simulink model "wiener"  (R2019b)
settings: Solver=VariableStepAuto  StartTime=0.0  StopTime=stopTime  RelTol=1e-3
InitFcn:
  | Init;
values from neighbouring files (symbols this model uses):
  Ts = 1/Fs    [Init.m]
libraries: simulink x2
settings Model: Creator=cb54103  LastModifiedBy=cb54103

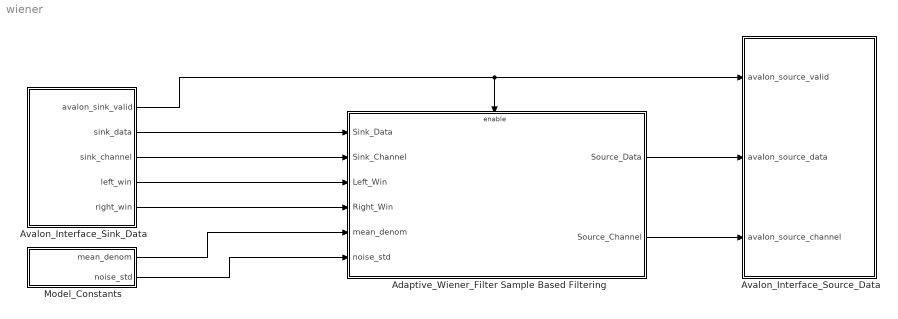
== system wiener ==
  Adaptive_Wiener_Filter Sample Based Filtering : Subsystem
  Avalon_Interface_Sink_Data : Subsystem
  Avalon_Interface_Source_Data : Subsystem
  Model_Constants : Subsystem
  wires:
  Adaptive_Wiener_Filter Sample Based Filtering/1(Source_Data) -> Avalon_Interface_Source_Data/2(avalon_source_data)
  Adaptive_Wiener_Filter Sample Based Filtering/2(Source_Channel) -> Avalon_Interface_Source_Data/3(avalon_source_channel)
  Avalon_Interface_Sink_Data/2(sink_data) -> Adaptive_Wiener_Filter Sample Based Filtering/1(Sink_Data)
  Avalon_Interface_Sink_Data/3(sink_channel) -> Adaptive_Wiener_Filter Sample Based Filtering/2(Sink_Channel)
  Avalon_Interface_Sink_Data/4(left_win) -> Adaptive_Wiener_Filter Sample Based Filtering/3(Left_Win)
  Avalon_Interface_Sink_Data/5(right_win) -> Adaptive_Wiener_Filter Sample Based Filtering/4(Right_Win)
  Avalon_Interface_Sink_Data/1(avalon_sink_valid) -> Adaptive_Wiener_Filter Sample Based Filtering/Enable, Avalon_Interface_Source_Data/1(avalon_source_valid)
  Model_Constants/1(mean_denom) -> Adaptive_Wiener_Filter Sample Based Filtering/5(mean_denom)
  Model_Constants/2(noise_std) -> Adaptive_Wiener_Filter Sample Based Filtering/6(noise_std)

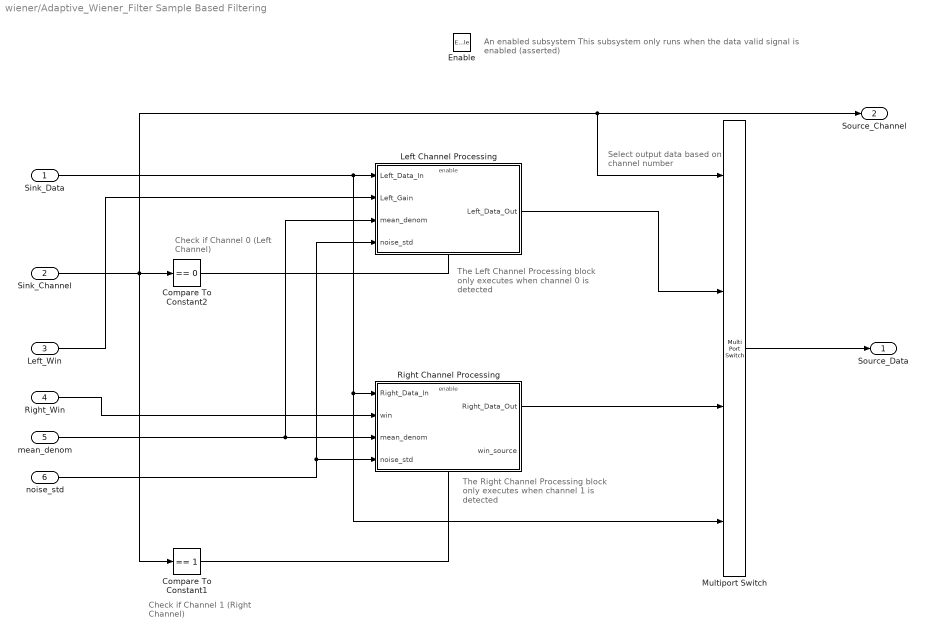
== system wiener/Adaptive_Wiener_Filter Sample Based Filtering ==
  note: The Left Channel Processing block
      | only executes when channel 0
      | is detected
  note: The Right Channel Processing block
      | only executes when channel 1
      | is detected
  note: Check if Channel 1
      | (Right Channel)
  note: Check if Channel 0
      | (Left Channel)
  note: Select output data
      | based on channel number
  note: An enabled subsystem
      | This subsystem only runs when the data valid signal is enabled (asserted)
  Sink_Data : Inport
  Sink_Channel : Inport  Port=2
  Left_Win : Inport  Port=3
  Right_Win : Inport  Port=4
  mean_denom : Inport  Port=5
  noise_std : Inport  Port=6
  Enable : EnablePort
  Compare To Constant1 : simulink/Logic and Bit Operations/Compare To Constant  relop===  const=1  OutDataTypeStr=boolean
  Compare To Constant2 : simulink/Logic and Bit Operations/Compare To Constant  relop===  const=0  OutDataTypeStr=boolean
  Left Channel Processing : Subsystem  TreatAsAtomicUnit=on
  Multiport Switch : MultiPortSwitch  DataPortOrder=Zero-based contiguous  zeroidx=on
  Right Channel Processing : Subsystem  TreatAsAtomicUnit=on
  Source_Data : Outport  InitialOutput=0  VectorParamsAs1DForOutWhenUnconnected=off
  Source_Channel : Outport  Port=2  InitialOutput=0  VectorParamsAs1DForOutWhenUnconnected=off
  wires:
  Left Channel Processing/1("Left_Data_Out ") -> Multiport Switch/2
  Multiport Switch/1 -> Source_Data/1
  Compare To Constant2/1 -> Left Channel Processing/Enable
  Right_Win/1 -> Right Channel Processing/2(win)
  Left_Win/1 -> Left Channel Processing/2(Left_Gain)
  Sink_Data/1 -> Multiport Switch/4, Right Channel Processing/1(Right_Data_In), Left Channel Processing/1(Left_Data_In)
  Right Channel Processing/1("Right_Data_Out ") -> Multiport Switch/3
  Sink_Channel/1 -> Source_Channel/1, Multiport Switch/1, Compare To Constant1/1, Compare To Constant2/1
  Compare To Constant1/1 -> Right Channel Processing/Enable
  mean_denom/1 -> Left Channel Processing/3(mean_denom), Right Channel Processing/3(mean_denom)
  noise_std/1 -> Left Channel Processing/4(noise_std), Right Channel Processing/4(noise_std)

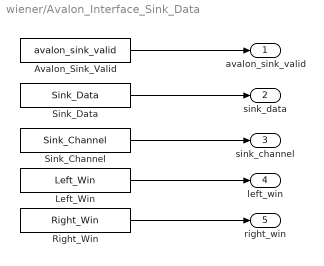
== system wiener/Avalon_Interface_Sink_Data ==
  Avalon_Sink_Valid : FromWorkspace  VariableName=avalon_sink_valid  SampleTime=Ts
  Left_Win : FromWorkspace  VariableName=Left_Win  SampleTime=Ts
  Right_Win : FromWorkspace  VariableName=Right_Win  SampleTime=Ts
  Sink_Channel : FromWorkspace  VariableName=Sink_Channel  SampleTime=Ts
  Sink_Data : FromWorkspace  VariableName=Sink_Data  SampleTime=Ts
  avalon_sink_valid : Outport  InitialOutput=0  VectorParamsAs1DForOutWhenUnconnected=off
  sink_data : Outport  Port=2  InitialOutput=0  VectorParamsAs1DForOutWhenUnconnected=off
  sink_channel : Outport  Port=3  InitialOutput=0  VectorParamsAs1DForOutWhenUnconnected=off
  left_win : Outport  Port=4  InitialOutput=0  VectorParamsAs1DForOutWhenUnconnected=off
  right_win : Outport  Port=5  InitialOutput=0  VectorParamsAs1DForOutWhenUnconnected=off
  wires:
  Sink_Channel/1 -> sink_channel/1
  Avalon_Sink_Valid/1 -> avalon_sink_valid/1
  Sink_Data/1 -> sink_data/1
  Left_Win/1 -> left_win/1
  Right_Win/1 -> right_win/1

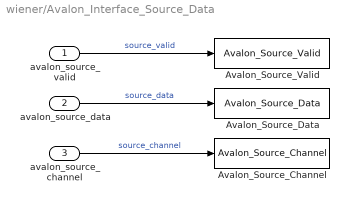
== system wiener/Avalon_Interface_Source_Data ==
  avalon_source_valid : Inport
  avalon_source_data : Inport  Port=2
  avalon_source_channel : Inport  Port=3
  Avalon_Source_Channel : ToWorkspace  VariableName=Avalon_Source_Channel  SaveFormat=Timeseries  SampleTime=-1
  Avalon_Source_Data : ToWorkspace  VariableName=Avalon_Source_Data  SaveFormat=Timeseries  SampleTime=-1
  Avalon_Source_Valid : ToWorkspace  VariableName=Avalon_Source_Valid  SaveFormat=Timeseries  SampleTime=-1
  wires:
  avalon_source_valid/1 -> Avalon_Source_Valid/1  "source_valid"
  avalon_source_data/1 -> Avalon_Source_Data/1  "source_data"
  avalon_source_channel/1 -> Avalon_Source_Channel/1  "source_channel"

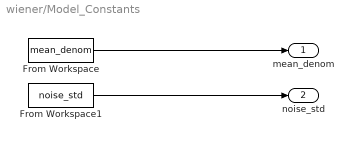
== system wiener/Model_Constants ==
  From Workspace : FromWorkspace  VariableName=mean_denom  SampleTime=Ts
  From Workspace1 : FromWorkspace  VariableName=noise_std  SampleTime=Ts
  mean_denom : Outport
  noise_std : Outport  Port=2
  wires:
  From Workspace/1 -> mean_denom/1
  From Workspace1/1 -> noise_std/1

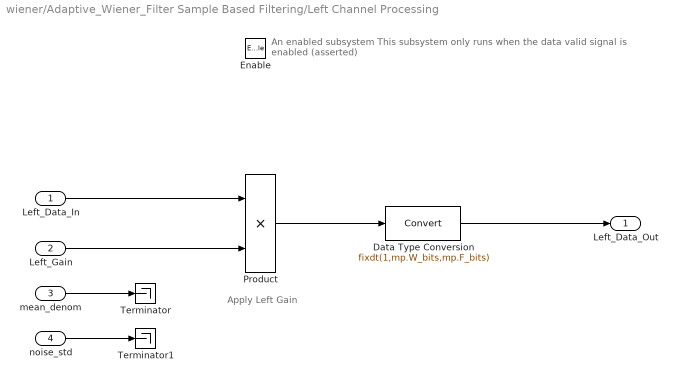
== system wiener/Adaptive_Wiener_Filter Sample Based Filtering/Left Channel Processing ==
  note: Apply Left Gain
  note: An enabled subsystem
      | This subsystem only runs when the data valid signal is enabled (asserted)
  Left_Data_In : Inport
  Left_Gain : Inport  Port=2
  mean_denom : Inport  Port=3
  noise_std : Inport  Port=4
  Enable : EnablePort
  Data Type Conversion : DataTypeConversion  OutDataTypeStr=fixdt(1,mp.W_bits,mp.F_bits)
  Product : Product
  Terminator : Terminator
  Terminator1 : Terminator
  "Left_Data_Out " : Outport  InitialOutput=0  VectorParamsAs1DForOutWhenUnconnected=off
  wires:
  Left_Data_In/1 -> Product/1
  Product/1 -> Data Type Conversion/1
  Data Type Conversion/1 -> "Left_Data_Out "/1
  Left_Gain/1 -> Product/2
  mean_denom/1 -> Terminator/1
  noise_std/1 -> Terminator1/1

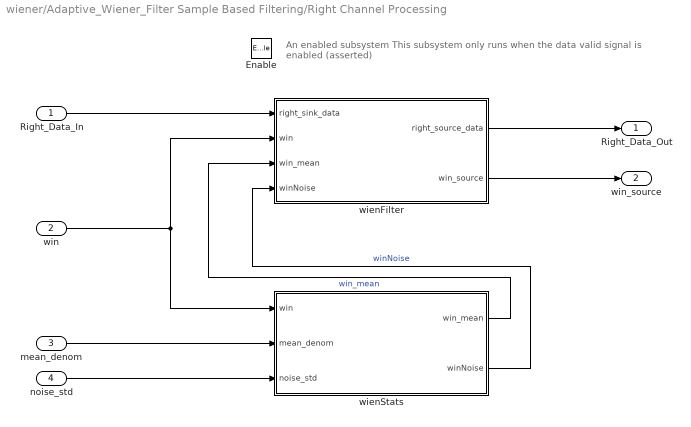
== system wiener/Adaptive_Wiener_Filter Sample Based Filtering/Right Channel Processing ==
  note: An enabled subsystem
      | This subsystem only runs when the data valid signal is enabled (asserted)
  Right_Data_In : Inport
  win : Inport  Port=2
  mean_denom : Inport  Port=3
  noise_std : Inport  Port=4
  Enable : EnablePort
  wienFilter : Subsystem
  wienStats : Subsystem
  "Right_Data_Out " : Outport  InitialOutput=0  VectorParamsAs1DForOutWhenUnconnected=off
  win_source : Outport  Port=2  InitialOutput=0  VectorParamsAs1DForOutWhenUnconnected=off
  wires:
  wienFilter/1(right_source_data) -> "Right_Data_Out "/1
  mean_denom/1 -> wienStats/2(mean_denom)
  noise_std/1 -> wienStats/3(noise_std)
  Right_Data_In/1 -> wienFilter/1(right_sink_data)
  win/1 -> wienFilter/2(win), wienStats/1(win)
  wienStats/1(win_mean) -> wienFilter/3(win_mean)  "win_mean"
  wienStats/2(winNoise) -> wienFilter/4(winNoise)  "winNoise"
  wienFilter/2(win_source) -> win_source/1

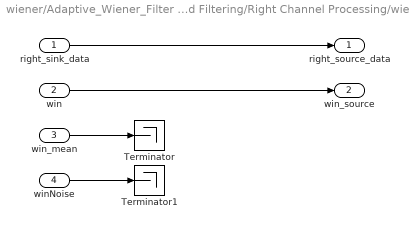
== system wiener/Adaptive_Wiener_Filter Sample Based Filtering/Right Channel Processing/wienFilter ==
  right_sink_data : Inport
  win : Inport  Port=2
  win_mean : Inport  Port=3
  winNoise : Inport  Port=4
  Terminator : Terminator
  Terminator1 : Terminator
  right_source_data : Outport
  win_source : Outport  Port=2
  wires:
  win_mean/1 -> Terminator/1
  winNoise/1 -> Terminator1/1
  win/1 -> win_source/1
  right_sink_data/1 -> right_source_data/1

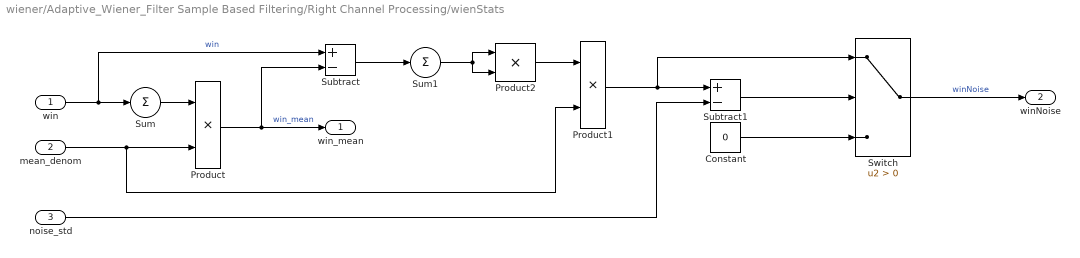
== system wiener/Adaptive_Wiener_Filter Sample Based Filtering/Right Channel Processing/wienStats ==
  win : Inport
  mean_denom : Inport  Port=2
  noise_std : Inport  Port=3
  Constant : Constant  Value=0  SampleTime=-1
  Product : Product
  Product1 : Product
  Product2 : Product
  Subtract : Sum  Inputs=+-
  Subtract1 : Sum  Inputs=+-
  Sum : Sum  Inputs=+
  Sum1 : Sum  Inputs=+
  Switch : Switch  Criteria=u2 > Threshold
  win_mean : Outport
  winNoise : Outport  Port=2
  wires:
  win/1 -> Subtract/1, Sum/1  "win"
  Sum/1 -> Product/1
  mean_denom/1 -> Product1/2, Product/2
  Product/1 -> Subtract/2, win_mean/1  "win_mean"
  Subtract/1 -> Sum1/1
  Sum1/1 -> Product2/1, Product2/2
  Product2/1 -> Product1/1
  noise_std/1 -> Subtract1/2
  Product1/1 -> Subtract1/1, Switch/1
  Subtract1/1 -> Switch/2
  Switch/1 -> winNoise/1  "winNoise"
  Constant/1 -> Switch/3
